simulink model "Edr"  (R2020b)
settings: configuration reference "gen_config" (kept outside this file)
undefined symbols (not defined in the file): Edr_nEdr, Edr_pwr_LossMap_AXIS, Edr_pwrElecEffEdr, Edr_pwrInverterLosses_MAP, Edr_pwrMachineLosses_MAP, Edr_pwrTotalLossesEdr, Edr_rpm_InvLossMap_AXIS, Edr_rpm_MachLossMap_AXIS, Edr_tq_MachLossMap_AXIS, Edr_tqEffEdr, Edr_wEdr
settings Model: DataDictionary=Hybrid_vehicle_update.sldd  SimulationMode=accelerator  Creator=Georg  LastModifiedBy=jy
settings ConfigSetRef: SourceName=gen_config

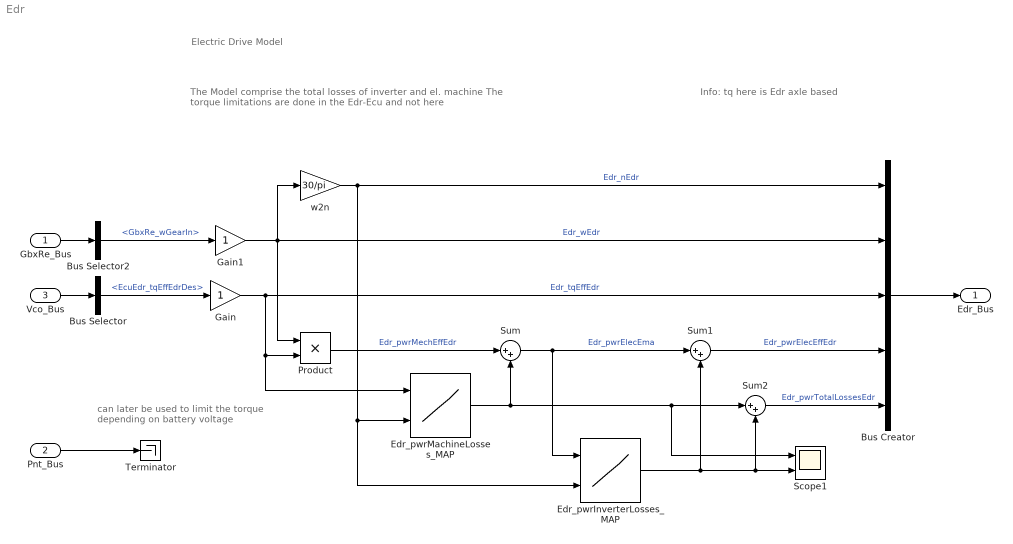
== system Edr ==
  note: Electric Drive Model
  note: can later be used to limit the torque
      | depending on battery voltage
  note: Info:
      | tq here is Edr axle based
  note: The Model comprise the total losses of inverter and el. machine
      | The torque limitations are done in the Edr-Ecu and not here
  GbxRe_Bus : Inport  OutDataTypeStr=Bus: GBXRE_BUS
  Pnt_Bus : Inport  Port=2  OutDataTypeStr=Bus: PNT_BUS
  Vco_Bus : Inport  Port=3  OutDataTypeStr=Bus: VCO_BUS
  Bus Creator : BusCreator  Inputs=Edr_nEdr,Edr_wEdr,Edr_tqEffEdr,Edr_pwrElecEffEdr,Edr_pwrTotalLossesEdr  OutDataTypeStr=Bus: EDR_BUS  NonVirtualBus=on
  Bus Selector : BusSelector  OutputSignals=EcuEdr_Bus.EcuEdr_tqEffEdrDes
  Bus Selector2 : BusSelector  OutputSignals=GbxRe_wGearIn
  Edr_pwrInverterLosses_MAP : Lookup_n-D  BreakpointsForDimension1=Edr_pwr_LossMap_AXIS  BreakpointsForDimension2=Edr_rpm_InvLossMap_AXIS  Table=Edr_pwrInverterLosses_MAP  ExtrapMethod=Clip  UseLastTableValue=on  InternalRulePriority=Speed  RndMeth=Simplest  InputSameDT=on
      settings: InputPortMap=u0,u1
  Edr_pwrMachineLosses_MAP : Lookup_n-D  BreakpointsForDimension1=Edr_tq_MachLossMap_AXIS  BreakpointsForDimension2=Edr_rpm_MachLossMap_AXIS  Table=Edr_pwrMachineLosses_MAP  ExtrapMethod=Clip  UseLastTableValue=on  InternalRulePriority=Speed  RndMeth=Simplest  InputSameDT=on
      settings: InputPortMap=u0,u1
  Gain : Gain
  Gain1 : Gain
  Product : Product
  Scope1 : Scope  NumInputPorts=2
  Sum : Sum  Inputs=|++
  Sum1 : Sum  Inputs=|++
  Sum2 : Sum  Inputs=|++
  Terminator : Terminator
  w2n : Gain  Gain=30/pi
  Edr_Bus : Outport  OutDataTypeStr=Bus: EDR_BUS  VectorParamsAs1DForOutWhenUnconnected=off
  wires:
  Gain/1 -> Edr_pwrMachineLosses_MAP/1, Product/2, Bus Creator/3  "Edr_tqEffEdr"
  Sum2/1 -> Bus Creator/5  "Edr_pwrTotalLossesEdr"
  Bus Creator/1 -> Edr_Bus/1
  Product/1 -> Sum/1  "Edr_pwrMechEffEdr"
  Sum/1 -> Sum1/1, Edr_pwrInverterLosses_MAP/1  "Edr_pwrElecEma"
  w2n/1 -> Bus Creator/1, Edr_pwrInverterLosses_MAP/2, Edr_pwrMachineLosses_MAP/2  "Edr_nEdr"
  Gain1/1 -> Bus Creator/2, w2n/1, Product/1  "Edr_wEdr"
  Bus Selector2/1 -> Gain1/1  "<GbxRe_wGearIn>"
  Vco_Bus/1 -> Bus Selector/1
  Bus Selector/1 -> Gain/1  "<EcuEdr_tqEffEdrDes>"
  Sum1/1 -> Bus Creator/4  "Edr_pwrElecEffEdr"
  Edr_pwrMachineLosses_MAP/1 -> Sum/2, Sum2/1, Scope1/1
  GbxRe_Bus/1 -> Bus Selector2/1
  Edr_pwrInverterLosses_MAP/1 -> Sum1/2, Sum2/2, Scope1/2
  Pnt_Bus/1 -> Terminator/1
